simulink model "simulink_5_1"  (R2015a)
settings: Solver=ode45  StartTime=0.0  StopTime=10.0  RelTol=1e-3
settings Model: Creator=Bojana Vasic  LastModifiedBy=Bojana Vasic

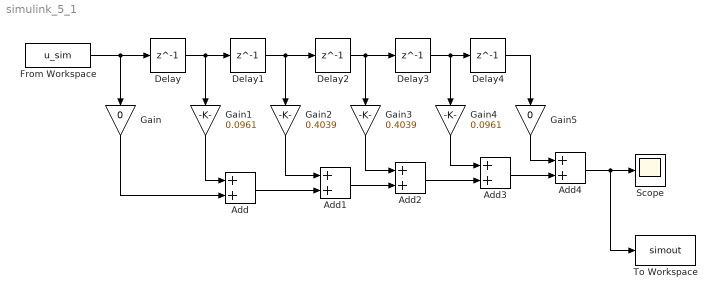
== system simulink_5_1 ==
  Add{,1..4} (5 alike) : Sum
  Delay{,1..4} (5 alike) : Delay  DelayLength=1
  From Workspace : FromWorkspace  VariableName=u_sim  SampleTime=1
  Gain : Gain  Gain=0
  Gain1 : Gain  Gain=0.0961
  Gain2 : Gain  Gain=0.4039
  Gain3 : Gain  Gain=0.4039
  Gain4 : Gain  Gain=0.0961
  Gain5 : Gain  Gain=0
  Scope : Scope
  To Workspace : ToWorkspace  VariableName=simout  SampleTime=-1
  wires:
  From Workspace/1 -> Gain/1, Delay/1
  Gain/1 -> Add/2
  Delay/1 -> Delay1/1, Gain1/1
  Gain1/1 -> Add/1
  Delay1/1 -> Delay2/1, Gain2/1
  Delay2/1 -> Delay3/1, Gain3/1
  Gain2/1 -> Add1/1
  Add/1 -> Add1/2
  Gain3/1 -> Add2/1
  Add1/1 -> Add2/2
  Delay3/1 -> Gain4/1, Delay4/1
  Add2/1 -> Add3/2
  Gain4/1 -> Add3/1
  Delay4/1 -> Gain5/1
  Gain5/1 -> Add4/1
  Add3/1 -> Add4/2
  Add4/1 -> To Workspace/1, Scope/1
